simulink model "Dynamic_Plant_Model"  (R2021a)
settings: Solver=VariableStepAuto  StartTime=0.0  StopTime=22  RelTol=1e-3
settings Model: Creator=User  LastModifiedBy=User

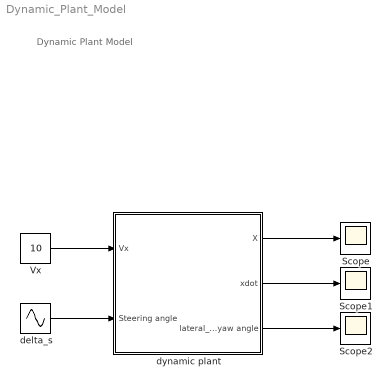
== system Dynamic_Plant_Model ==
  note: Dynamic Plant Model
  Scope : Scope
  Scope1 : Scope
  Scope2 : Scope
  Vx : Constant  Value=10
  delta_s : Sin  Amplitude=0.4  SampleTime=0
  dynamic plant : Subsystem
  wires:
  Vx/1 -> dynamic plant/1(Vx)
  delta_s/1 -> dynamic plant/2(Steering angle)
  dynamic plant/1(X) -> Scope/1
  dynamic plant/2(xdot) -> Scope1/1
  dynamic plant/3("lateral_pos & yaw angle  ") -> Scope2/1

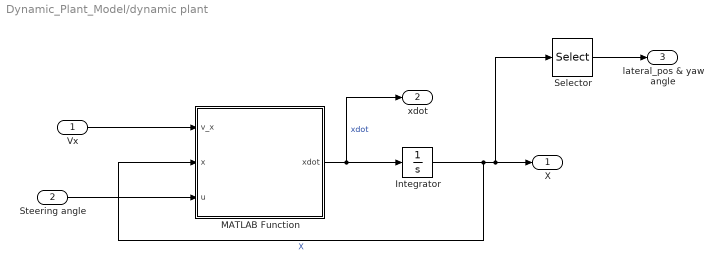
== system Dynamic_Plant_Model/dynamic plant ==
  Vx : Inport
  Steering angle : Inport  Port=2
  Integrator : Integrator
  MATLAB Function : MATLAB Function  TreatAsAtomicUnit=on
  Selector : Selector  InputPortWidth=4  IndexOptions=Index vector (dialog)  Indices=[1 3]  OutputSizes=1
  X : Outport
  xdot : Outport  Port=2
  "lateral_pos & yaw angle  " : Outport  Port=3
  wires:
  Steering angle/1 -> MATLAB Function/3(u)
  Vx/1 -> MATLAB Function/1(v_x)
  MATLAB Function/1(xdot) -> xdot/1, Integrator/1  "xdot"
  Integrator/1 -> MATLAB Function/2(x), Selector/1, X/1  "X"
  Selector/1 -> "lateral_pos & yaw angle  "/1

== matlab function Dynamic_Plant_Model/dynamic plant/MATLAB Function ==
  data: v_x input; x input; u input; xdot output
function xdot = fcn(v_x,x,u)

%% Model parameters
m = 1140;
I_z = 1436.24;%kgm2
l_f = 1.165;
l_r = 1.165;
c_f = 155494.663;% cf for front tire
c_r = 155494.663;% cr for front tire

%% Continous plant model in state space form
A = [0 1 0 0;
    0 -2*(c_f+c_r)/(m*v_x) 0 -2*(l_f*c_f+l_r*c_r)/(m*v_x) - v_x;
    0 0 0 1;
    0 2*(l_r*c_r-l_f*c_f)/(I_z*v_x) 0 -2*(l_r^2*c_r-l_f^2*c_f)/(I_z*v_x)];

B = [0;
    2*c_f/m;
    0;
    2*l_f*c_f/I_z];

C = [1 0 0 0;
    0 1 0 0];

D = [0];

xdot = A*x +B*u;
y = C*x + D*u;
end
